simulink model "Uebung11_2016a"  (R2016a)
settings: Solver=ode4  SolverMode=SingleTasking  StartTime=0.0  StopTime=100  FixedStep=0.1  RelTol=1e-3
values from neighbouring files (symbols this model uses):
  c = 500    [Uebung1.m]    (also in Uebung11.m = 5000)
  d = 5    [Uebung1.m]    (also in Uebung11.m = 0.01)
  g = 9.81    [Uebung1.m]
  m = 10    [Uebung1.m]    (also in Uebung11.m)
settings Model: Creator=Jason  LastModifiedBy=Jason
settings DebuggingCC: SFUnexpectedBacktrackingDiag=error  SFNoUnconditionalDefaultTransitionDiag=error
settings GRTTargetCC: TargetLangStandard=C99 (ISO)  GeneratePreprocessorConditionals=Use local settings
settings ConfigComp: CovMetricSettings=dwe  CovHtmlReporting=off  CovSaveCumulativeToWorkspaceVar=off  CovSaveSingleToWorkspaceVar=off  CovExternalEMLEnable=on

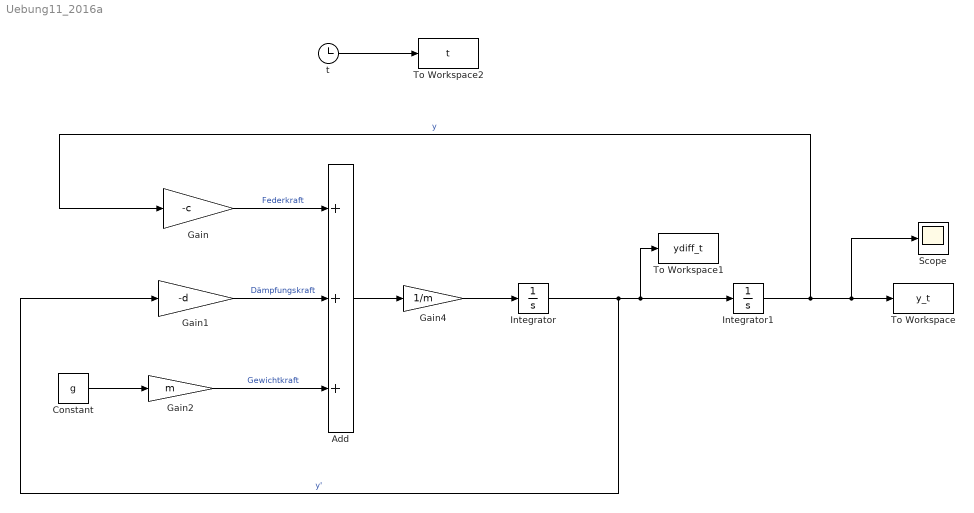
== system Uebung11_2016a ==
  Add : Sum  Inputs=+++
  Constant : Constant  Value=g
  Gain : Gain  Gain=-c
  Gain1 : Gain  Gain=-d
  Gain2 : Gain  Gain=m
  Gain4 : Gain  Gain=1/m
  Integrator : Integrator
  Integrator1 : Integrator
  Scope : Scope
  To Workspace : ToWorkspace  VariableName=y_t  SampleTime=-1
  To Workspace1 : ToWorkspace  VariableName=ydiff_t  SampleTime=-1
  To Workspace2 : ToWorkspace  VariableName=t  SampleTime=-1
  t : Clock
  wires:
  Integrator/1 -> Gain1/1, To Workspace1/1, Integrator1/1  "y'"
  Integrator1/1 -> Gain/1, Scope/1, To Workspace/1  "y"
  t/1 -> To Workspace2/1
  Gain2/1 -> Add/3  "Gewichtkraft"
  Gain/1 -> Add/1  "Federkraft"
  Gain1/1 -> Add/2  "Dämpfungskraft"
  Add/1 -> Gain4/1
  Gain4/1 -> Integrator/1
  Constant/1 -> Gain2/1
